simulink model "full_vehicle_sim"  (R2025b)
settings: Solver=VariableStepAuto  StartTime=0.0  StopTime=500  RelTol=1e-3
libraries: fl_lib x9, nesl_utility x5, SimscapeFluids_lib x2
(part 3 of 3)

== matlab function full_vehicle_sim/Vehicle Sim/OX Side Tanks/MATLAB Function ==
  data: mdot_l input; P_out output; rho_l_out output; P_in input; rho_g_in input; rho_g_out output; dt input; fill output
function [P_out, rho_l_out, rho_g_out, fill] = tank_model( ...
    mdot_l, P_in, rho_g_in, dt)

% --- Persistent States ---
persistent m_l m_g U_g V_total P

if isempty(m_l)
    % --- INITIAL CONDITIONS ---
    V_total = 0.01;     % m^3 (10 L tank)
    m_l = 5.0;          % kg liquid
    m_g = 0.05;         % kg ullage gas
    U_g = 5e4;          % J gas internal energy
    P = 5e5;            % Pa initial pressure
end

% --- CONSTANTS ---
rho_l = 1000;          % liquid density (kg/m^3)
R = 296.8;             % nitrogen gas constant
cv = 743;              % nitrogen cv
gamma = 1.4;

CdA = 1e-5;            % flow coefficient (tune this)
T_in = 300;            % inlet gas temperature (K)

% --- LIQUID VOLUME ---
V_l = m_l / rho_l;
V_g = V_total - V_l;

if V_g < 1e-6
    V_g = 1e-6;
end

% --- GAS STATE (from tank energy) ---
T_g = U_g / (m_g * cv);
rho_g = m_g / V_g;

% --- TANK PRESSURE (EOS) ---
P = rho_g * R * T_g;

% --- FLOW USING INPUT DENSITY ---
rho_in = rho_g_in;

critical_ratio = (2/(gamma+1))^(gamma/(gamma-1));

if P_in > P
    if (P / P_in) < critical_ratio
        % --- CHOKED FLOW ---
        mdot_g = CdA * P_in * sqrt(gamma/(R*T_in)) * ...
            (2/(gamma+1))^((gamma+1)/(2*(gamma-1)));
    else
        % --- SUBSONIC FLOW ---
        mdot_g = CdA * sqrt(2 * rho_in * (P_in - P));
    end
else
    mdot_g = 0;
end

% --- EXPANSION WORK (gas loses energy when expanding) ---
vol_change_rate = -(mdot_l / rho_l);
work = P * vol_change_rate;

% --- MASS UPDATE ---
m_l = m_l + mdot_l * dt;
m_g = m_g + mdot_g * dt;

% --- ENERGY UPDATE (gas only) ---
U_g = U_g - work * dt;

% --- SAFETY LIMITS ---
if m_l < 1e-6; m_l = 1e-6; end
if m_g < 1e-6; m_g = 1e-6; end

% --- RECOMPUTE VOLUMES ---
V_l = m_l / rho_l;
V_g = V_total - V_l;

if V_g < 1e-6
    V_g = 1e-6;
end

% --- FINAL STATE UPDATE ---
rho_g = m_g / V_g;
T_g = U_g / (m_g * cv);
P = rho_g * R * T_g;

% --- OUTPUTS ---
P_out = P;
rho_l_out = rho_l;
rho_g_out = rho_g;
fill = V_l / V_total;

end
